simulink model "test_SF"  (R2020b)
settings: Solver=VariableStepAuto  StartTime=0.0  StopTime=20  RelTol=1e-3
undefined symbols (not defined in the file): C, K_SF
settings Model: Creator=10911  LastModifiedBy=10911

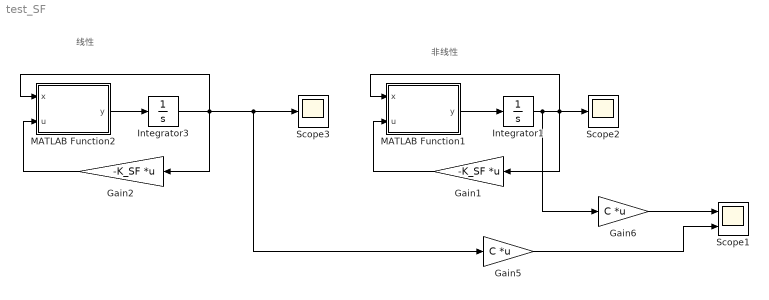
== system test_SF ==
  note: 线性
  note: 非线性
  Gain1 : Gain  Gain=-K_SF  Multiplication=Matrix(K*u)
  Gain2 : Gain  Gain=-K_SF  Multiplication=Matrix(K*u)
  Gain5 : Gain  Gain=C  Multiplication=Matrix(K*u)
  Gain6 : Gain  Gain=C  Multiplication=Matrix(K*u)
  Integrator1 : Integrator  InitialCondition=[0,0,0.3,0]
  Integrator3 : Integrator  InitialCondition=[0;0;0.1;0]
  MATLAB Function1 : MATLAB Function  TreatAsAtomicUnit=on
  MATLAB Function2 : MATLAB Function  TreatAsAtomicUnit=on
  Scope1 : Scope  NumInputPorts=2
  Scope2 : Scope
  Scope3 : Scope
  wires:
  Gain2/1 -> MATLAB Function2/2(u)
  MATLAB Function1/1(y) -> Integrator1/1
  Integrator1/1 -> Gain6/1, Gain1/1, MATLAB Function1/1(x), Scope2/1
  Gain1/1 -> MATLAB Function1/2(u)
  Integrator3/1 -> Gain2/1, MATLAB Function2/1(x), Gain5/1, Scope3/1
  MATLAB Function2/1(y) -> Integrator3/1
  Gain6/1 -> Scope1/1
  Gain5/1 -> Scope1/2

== matlab function test_SF/MATLAB Function2 ==
  data: x input; y output; u input
function y = fcn(x,u)

dx1 = x(2);
dx2 = -x(3)+u;
dx3 = x(4);
dx4 = 22*x(3)-2*u;

y = [dx1;dx2;dx3;dx4];

== matlab function test_SF/MATLAB Function1 ==
  data: x input; y output; u input
function y = fcn(x,u)
M = 1;
m = 0.1;
l = 0.5;
g = 9.8;
x1=x(1);
x2=x(2);
x3=x(3);
x4=x(4);

dx1 = x2;
dx2 =(u + m*l*x4*x4*sin(x3) - m*g*sin(x3)*cos(x3))/(M + m - m*cos(x3)*cos(x3));
dx3 = x4;
dx4 =(-u*cos(x3) + (M+m)*g*sin(x3) - m*l*x4*x4*sin(x3)*cos(x3))/((M+m)*l - m*l*cos(x3)*cos(x3));
y = [dx1;dx2;dx3;dx4];
